simulink model "Thermal_Network_Model"  (R2022b)
settings: Solver=VariableStepAuto  StartTime=0.0  StopTime=24*3600*1  FixedStep=1  RelTol=1e-3  AbsTol=1e-3  EnableMultiTasking=on
InitFcn:
  | % Roof
  | roofArea =  2* (widHouse/(2*cos(pitRoof))*lenHouse);
  | 
  | %Rooms
  | %% Room 1
  | area_window_room1 = 3 * 1 *1;
  | area_wall_room1 = (lenHouse*3/5 *htHouse+widHouse*2/3*htHouse) - area_window_room1;
  | area_roof_room1 = roofArea/4;
  | 
  | %% Room 2
  | area_window_room2 = 2 * 1 *1;
  | area_wall_room2 = (lenHouse*3/5*htHouse+widHouse/3*htHouse) - area_window_room2;
  | area_roof_room2 = roofArea/4;
  | 
  | %% Room 3
  | area_window_room3 =2* 1 *1;
  | area_wall_room3 = (lenHouse*2/5*htHouse+widHouse*2/3*htHouse) - area_window_room3;
  | area_roof_room3 = roofArea/4;
  | 
  | %% Room 4
  | area_window_room4 = 2 * 1 *1;
  | area_wall_room4 = (lenHouse*2/5*htHouse+widHouse/3*htHouse) - area_window_room4;
  | area_roof_room4 = roofArea/4;
  | 
  | % Cost estimation
  | % Assume the cost of natural gas is $8.50 per thousand cubic feet (Mcf): $8.50 per 1000 cf
  | % cost = $8.50/(1000 * 0.02831) m^3
  | cost = 8.50/(1000 * 0.02831);
  | % Natural gas density ~ 0.9 kg/m^3
  | NG_density = 0.9;
values from neighbouring files (symbols this model uses):
  airDensity = 1.025    [Model_inputs.m]
  htHouse = 2.6    [Model_inputs.m]
  LCavity = 0.014    [Model_inputs.m]
  lenHouse = 15    [Model_inputs.m]
  load = struct()    [Model_inputs.m]
  LRoof = 0.2    [Model_inputs.m]
  LWall = 0.25    [Model_inputs.m]
  LWindow = 0.004    [Model_inputs.m]
  panel = struct()    [Model_inputs.m]
  pipe = struct()    [Model_inputs.m]
  pitRoof = 40/180/pi    (= 0.0707355302631)    [Model_inputs.m]
  roofDensity = 2440    [Model_inputs.m]
  tank = struct()    [Model_inputs.m]
  temp_initial = 20    [Model_inputs.m]
  wallDensity = 2400    [Model_inputs.m]
  widHouse = 8    [Model_inputs.m]
  windowDensity = 2500    [Model_inputs.m]
libraries: fl_lib x188, nesl_utility x51, SimscapeFluids_lib x14, fuzblock x6, ee_lib x1
(part 2 of 4)

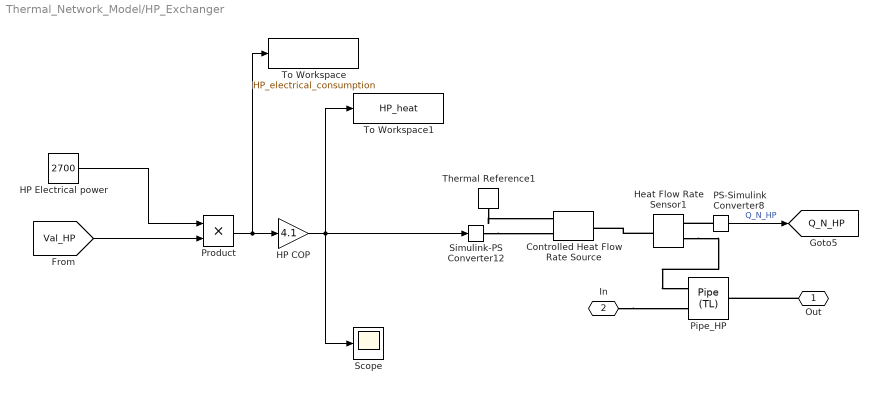
== system Thermal_Network_Model/HP_Exchanger ==
  Controlled Heat Flow Rate Source : fl_lib/Thermal/Thermal Sources/Controlled Heat Flow Rate Source
  HP COP : Gain  Gain=4.1
  HP Electrical power : Constant  Value=2700
  Heat Flow Rate Sensor1 : fl_lib/Thermal/Thermal Sensors/Heat Flow Rate Sensor
  PS-Simulink Converter8 : nesl_utility/PS-Simulink Converter  PhysicalDomain=network_engine_domain  SubClassName=ps_output  LeftPortType=input  RightPortType=output  PseudoPeriodic=off  Frequencies=[]  VectorFormat=1-D array  Unit=inherit  AffineConversion=off
  Pipe_HP : fl_lib/Thermal Liquid/Elements/Pipe (TL)  length=pipe.length m  area=pipe.area m^2  Dh=pipe.Dh m  length_add=pipe.length_add m  roughness=pipe.roughness m  Re_lam=pipe.Re_lam  Re_tur=pipe.Re_tur  shape_factor=pipe.shape_factor  Nu_lam=pipe.Nu_lam  dynamic_compressibility=simscape.enum.onoff.off  inertia=simscape.enum.onoff.off  p0=0.101325 MPa  T0=panel.initial.Tw0 K  mdot0=0 kg/s
  Product : Product
  Scope : Scope
  Simulink-PS Converter12 : nesl_utility/Simulink-PS Converter  PhysicalDomain=network_engine_domain  SubClassName=ps_input  LeftPortType=input  RightPortType=output  PseudoPeriodic=off  Frequencies=[]  NoiseDistribution=none  NoiseParameters=[]  Unit=1  AffineConversion=off  FilteringAndDerivatives=provide  SimscapeFilterOrder=1  InputFilterTimeConstant=0.001  UdotUserProvided=0
  Thermal Reference1 : fl_lib/Thermal/Thermal Elements/Thermal Reference
  To Workspace : ToWorkspace  VariableName=HP_electrical_consumption  SaveFormat=Timeseries  SampleTime=60
  To Workspace1 : ToWorkspace  VariableName=HP_heat  SaveFormat=Timeseries  SampleTime=60
  Out : PMIOPort  Side=Left
  In : PMIOPort  Port=2  Side=Right
  tag scope: Q_N_HP=global
  wires:
  PS-Simulink Converter8/1 -> [Q_N_HP]  "Q_N_HP"
  Product/1 -> To Workspace/1, HP COP/1
  [Val_HP] -> Product/2
  HP COP/1 -> Simulink-PS Converter12/1, Scope/1, To Workspace1/1
  HP Electrical power/1 -> Product/1
  connections:
  Heat Flow Rate Sensor1/RConn2 -- Pipe_HP/LConn2
  Thermal Reference1/LConn1 -- Controlled Heat Flow Rate Source/RConn2
  Heat Flow Rate Sensor1/LConn1 -- Controlled Heat Flow Rate Source/LConn1
  PS-Simulink Converter8/LConn1 -- Heat Flow Rate Sensor1/RConn1
  Simulink-PS Converter12/RConn1 -- Controlled Heat Flow Rate Source/RConn1
  Out/RConn1 -- Pipe_HP/RConn1
  In/RConn1 -- Pipe_HP/LConn1

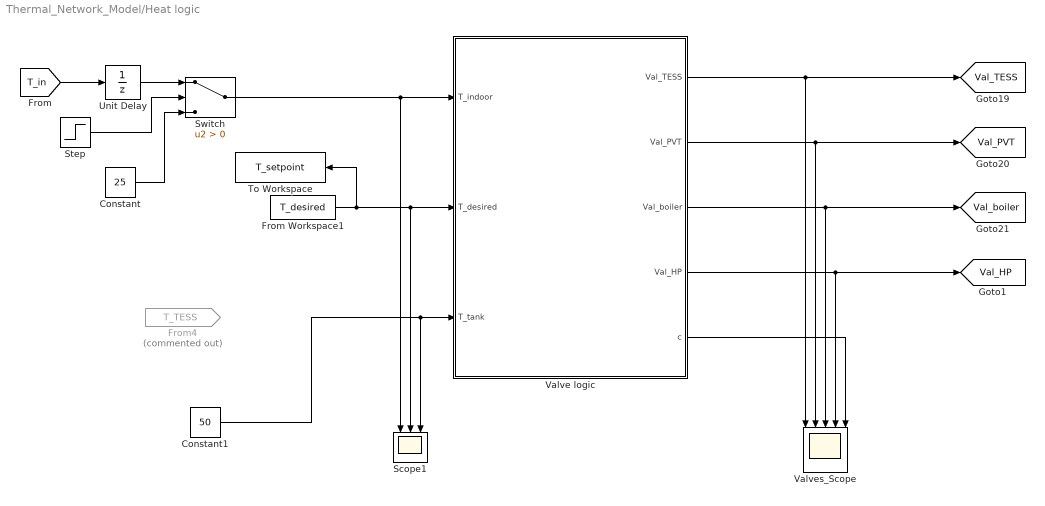
== system Thermal_Network_Model/Heat logic ==
  Constant : Constant  Value=25
  Constant1 : Constant  Value=50
  From Workspace1 : FromWorkspace  VariableName=T_desired
  From4 : From  Commented=on  GotoTag=T_TESS  TagVisibility=global
  Scope1 : Scope  NumInputPorts=3
  Step : Step  Time=3600  SampleTime=0
  Switch : Switch  Criteria=u2 > Threshold  SaturateOnIntegerOverflow=off  InputSameDT=off
  To Workspace : ToWorkspace  VariableName=T_setpoint  SaveFormat=Timeseries  SampleTime=-1
  Unit Delay : UnitDelay  SampleTime=-1  HasFrameUpgradeWarning=on
  Valve logic : MATLAB Function  TreatAsAtomicUnit=on
  Valves_Scope : Scope  NumInputPorts=5
  tag scope: Val_HP=global, Val_PVT=global, Val_TESS=global, Val_boiler=global
  wires:
  From Workspace1/1 -> To Workspace/1, Scope1/2, Valve logic/2(T_desired)
  Valve logic/1(Val_TESS) -> [Val_TESS], Valves_Scope/1
  Valve logic/2(Val_PVT) -> [Val_PVT], Valves_Scope/2
  Valve logic/3(Val_boiler) -> [Val_boiler], Valves_Scope/3
  Valve logic/4(Val_HP) -> [Val_HP], Valves_Scope/4
  Constant/1 -> Switch/3
  Step/1 -> Switch/2
  Switch/1 -> Scope1/1, Valve logic/1(T_indoor)
  [T_in] -> Unit Delay/1
  Unit Delay/1 -> Switch/1
  Valve logic/5(c) -> Valves_Scope/5
  Constant1/1 -> Valve logic/3(T_tank), Scope1/3

== system Thermal_Network_Model/House thermal network1 ==
  T_atm : Inport
  Indoor average temperature : Subsystem
  Radiator1 : Subsystem
      mask Display: disp('Radiator')
  Radiator2 : Subsystem
      mask Display: disp('Radiator')
  Radiator3 : Subsystem
      mask Display: disp('Radiator')
  Radiator4 : Subsystem
      mask Display: disp('Radiator')
  Room 1 : Subsystem  Tag=PublishSubsystem
      mask Display: disp('Room 1')
  Room 2 : Subsystem  Tag=PublishSubsystem
      mask Display: disp('Room 2')
  Room 3 : Subsystem  Tag=PublishSubsystem
      mask Display: disp('Room 3')
  Room 4 : Subsystem  Tag=PublishSubsystem
      mask Display: disp('Room 4')
  In : PMIOPort  Side=Left
  Out : PMIOPort  Port=2  Side=Left
  T_avg : Outport  VectorParamsAs1DForOutWhenUnconnected=off
  wires:
  T_atm/1 -> Room 1/1(Tatm), Room 2/1(Tatm), Room 3/1(Tatm), Room 4/1(Tatm)
  Indoor average temperature/1(T_avg) -> T_avg/1
  Room 2/1(Troom2) -> Indoor average temperature/3(T2)
  Room 4/1(Troom4) -> Indoor average temperature/1(T4)
  Room 3/1(Troom3) -> Indoor average temperature/2(T3)
  Room 1/1(Troom1) -> Indoor average temperature/4(T1)
  connections:
  Room 1/LConn1 -- Radiator1/LConn2
  Room 4/LConn1 -- Radiator4/LConn2
  Room 2/LConn1 -- Radiator2/LConn2
  Room 3/LConn1 -- Radiator3/LConn2
  Radiator1/RConn1 -- Out/RConn1 -- Radiator4/RConn1 -- Radiator3/RConn1 -- Radiator2/RConn1
  Radiator3/LConn1 -- Radiator2/LConn1 -- In/RConn1 -- Radiator1/LConn1 -- Radiator4/LConn1

== system Thermal_Network_Model/Network_Measures ==
  Absolute Reference (TL)2 : fl_lib/Thermal Liquid/Elements/Absolute Reference (TL)
  Density : Gain  Gain=1000
  PS-Simulink Converter5 : nesl_utility/PS-Simulink Converter  PhysicalDomain=network_engine_domain  SubClassName=ps_output  LeftPortType=input  RightPortType=output  PseudoPeriodic=off  Frequencies=[]  VectorFormat=1-D array  Unit=inherit  AffineConversion=off
  PS-Simulink Converter6 : nesl_utility/PS-Simulink Converter  PhysicalDomain=network_engine_domain  SubClassName=ps_output  LeftPortType=input  RightPortType=output  PseudoPeriodic=off  Frequencies=[]  VectorFormat=1-D array  Unit=inherit  AffineConversion=off
  PS-Simulink Converter7 : nesl_utility/PS-Simulink Converter  PhysicalDomain=network_engine_domain  SubClassName=ps_output  LeftPortType=input  RightPortType=output  PseudoPeriodic=off  Frequencies=[]  VectorFormat=1-D array  Unit=inherit  AffineConversion=off
  Pressure & Temperature Sensor (TL)2 : fl_lib/Thermal Liquid/Sensors/Pressure & Temperature Sensor (TL)
      settings: InternalSimscapePortConfiguration="{\"Bottom\":[],\"Left\":[{\"id\":\"A\",\"label\":\"A\",\"type\":\"foundation.thermal_liquid.thermal_liquid\"}],\"Right\":[{\"id\":\"B\",\"label\":\"B\",\"type\":\"foundation.thermal_liquid.thermal_liquid\"},{\"id\":\"P\",\"label\":\"P\",\"type\":\"output\"},{\"id\":\"T\",\"label\":\"T\",\"type\":\"output\"}],\"Top\":[]}"
  Volumetric Flow Rate Sensor (TL)1 : fl_lib/Thermal Liquid/Sensors/Volumetric Flow Rate Sensor (TL)
      settings: InternalSimscapePortConfiguration="{\"Bottom\":[],\"Left\":[{\"id\":\"A\",\"label\":\"A\",\"type\":\"foundation.thermal_liquid.thermal_liquid\"}],\"Right\":[{\"id\":\"B\",\"label\":\"B\",\"type\":\"foundation.thermal_liquid.thermal_liquid\"},{\"id\":\"V\",\"label\":\"V\",\"type\":\"output\"}],\"Top\":[]}"
  Out : PMIOPort  Side=Left
  In : PMIOPort  Port=2  Side=Right
  tag scope: P_Network=global, T_Network=global, massflow_Network=global
  wires:
  PS-Simulink Converter5/1 -> Density/1
  PS-Simulink Converter7/1 -> [P_Network]  "P_Network"
  Density/1 -> [massflow_Network]  "massflow_Network"
  PS-Simulink Converter6/1 -> [T_Network]  "T_Network"
  connections:
  Absolute Reference (TL)2/LConn1 -- Pressure & Temperature Sensor (TL)2/RConn1
  PS-Simulink Converter6/LConn1 -- Pressure & Temperature Sensor (TL)2/RConn3
  Volumetric Flow Rate Sensor (TL)1/RConn1 -- Out/RConn1 -- Pressure & Temperature Sensor (TL)2/LConn1
  PS-Simulink Converter5/LConn1 -- Volumetric Flow Rate Sensor (TL)1/RConn2
  PS-Simulink Converter7/LConn1 -- Pressure & Temperature Sensor (TL)2/RConn2
  In/RConn1 -- Volumetric Flow Rate Sensor (TL)1/LConn1

== system Thermal_Network_Model/Network_Pump ==
  Angular Velocity Source : fl_lib/Mechanical/Mechanical Sources/Ideal Angular Velocity Source
  Constant : Constant
  Fixed-Displacement Pump (TL) : SimscapeFluids_lib/Thermal Liquid/Pumps & Motors/Fixed-Displacement Pump (TL)  loss_spec=1  displacement=2e-5 m^3/rad  omega_nominal=150 rad/s  p_nominal=1 bar  mu_nominal=0.9 cP  vol_eff_nominal=0.92  mech_eff_nominal=0.88  no_load_torque=0.05 N*m  p_diff_eff_TLU=[0.1, 1, 2.55] MPa  omega_eff_TLU=[25, 50, 100, 200, 300, 400] rad/s  vol_eff_TLU=[0.816, 0.908, 0.954, 0.977, 0.981, 0.984; 0.325, 0.663, 0.831, 0.916, 0.925, 0.946; 0.137, 0.568, 0.78, 0.892, 0.893, 0.910]  mech_eff_TLU=[0.996, 0.996, 0.996, 0.996, 0.996, 0.996; 0.988, 0.989, 0.989, 0.989, 0.989, 0.990; 0.981, 0.981, 0.982, 0.982, 0.983, 0.984]  p_diff_loss_TLU=[.1, 1, 2] MPa  omega_loss_TLU=[25, 50, 100, 200, 300, 400] rad/s  vol_loss_TLU=[.023, .023, .023, .023, .0285, .032; .0844, .0842, .0845, .084, .1125, .108; .1079, .108, .11, .108, .1605, .18] * 1e-3 m^3/s  mech_loss_TLU=[.002, .002, .002, .002, .002, .002; .0607, .0556, .0556, .0556, .0556, .0505; .1937, .1937, .1833, .1833, .1729, .1626] N*m  vol_eff_min=1e-3  vol_eff_max=1  mech_eff_min=1e-3  mech_eff_max=1  pressure_threshold=1e-3 MPa  omega_threshold=10 rad/s  area=0.01 m^2  quadrant_check=0  pump_mode_check=simscape.enum.assert.action.none
  Mechanical Rotational Reference : fl_lib/Mechanical/Rotational Elements/Mechanical Rotational Reference
  Mechanical Rotational Reference1 : fl_lib/Mechanical/Rotational Elements/Mechanical Rotational Reference
  Product : Product
  Simulink-PS Converter : nesl_utility/Simulink-PS Converter  PhysicalDomain=network_engine_domain  SubClassName=ps_input  LeftPortType=input  RightPortType=output  PseudoPeriodic=off  Frequencies=[]  NoiseDistribution=none  NoiseParameters=[]  Unit=rpm  AffineConversion=off  FilteringAndDerivatives=zero  SimscapeFilterOrder=1  InputFilterTimeConstant=0.001  UdotUserProvided=1
  speed : Constant  Value=150*30/pi
  In : PMIOPort  Side=Left
  Out : PMIOPort  Port=2  Side=Right
  wires:
  Constant/1 -> Product/1
  Product/1 -> Simulink-PS Converter/1
  speed/1 -> Product/2
  connections:
  Out/RConn1 -- Fixed-Displacement Pump (TL)/LConn2
  Fixed-Displacement Pump (TL)/LConn1 -- In/RConn1
  Simulink-PS Converter/RConn1 -- Angular Velocity Source/RConn1
  Mechanical Rotational Reference1/LConn1 -- Angular Velocity Source/RConn2
  Mechanical Rotational Reference/LConn1 -- Fixed-Displacement Pump (TL)/RConn2
  Angular Velocity Source/LConn1 -- Fixed-Displacement Pump (TL)/RConn1

== system Thermal_Network_Model/Network_Pump1 ==
  Angular Velocity Source : fl_lib/Mechanical/Mechanical Sources/Ideal Angular Velocity Source
  Constant : Constant
  Fixed-Displacement Pump (TL) : SimscapeFluids_lib/Thermal Liquid/Pumps & Motors/Fixed-Displacement Pump (TL)  loss_spec=1  displacement=2e-5 m^3/rad  omega_nominal=150 rad/s  p_nominal=1 bar  mu_nominal=0.9 cP  vol_eff_nominal=0.92  mech_eff_nominal=0.88  no_load_torque=0.05 N*m  p_diff_eff_TLU=[0.1, 1, 2.55] MPa  omega_eff_TLU=[25, 50, 100, 200, 300, 400] rad/s  vol_eff_TLU=[0.816, 0.908, 0.954, 0.977, 0.981, 0.984; 0.325, 0.663, 0.831, 0.916, 0.925, 0.946; 0.137, 0.568, 0.78, 0.892, 0.893, 0.910]  mech_eff_TLU=[0.996, 0.996, 0.996, 0.996, 0.996, 0.996; 0.988, 0.989, 0.989, 0.989, 0.989, 0.990; 0.981, 0.981, 0.982, 0.982, 0.983, 0.984]  p_diff_loss_TLU=[.1, 1, 2] MPa  omega_loss_TLU=[25, 50, 100, 200, 300, 400] rad/s  vol_loss_TLU=[.023, .023, .023, .023, .0285, .032; .0844, .0842, .0845, .084, .1125, .108; .1079, .108, .11, .108, .1605, .18] * 1e-3 m^3/s  mech_loss_TLU=[.002, .002, .002, .002, .002, .002; .0607, .0556, .0556, .0556, .0556, .0505; .1937, .1937, .1833, .1833, .1729, .1626] N*m  vol_eff_min=1e-3  vol_eff_max=1  mech_eff_min=1e-3  mech_eff_max=1  pressure_threshold=1e-3 MPa  omega_threshold=10 rad/s  area=0.01 m^2  quadrant_check=0  pump_mode_check=simscape.enum.assert.action.none
  Mechanical Rotational Reference : fl_lib/Mechanical/Rotational Elements/Mechanical Rotational Reference
  Mechanical Rotational Reference1 : fl_lib/Mechanical/Rotational Elements/Mechanical Rotational Reference
  Product : Product
  Simulink-PS Converter : nesl_utility/Simulink-PS Converter  PhysicalDomain=network_engine_domain  SubClassName=ps_input  LeftPortType=input  RightPortType=output  PseudoPeriodic=off  Frequencies=[]  NoiseDistribution=none  NoiseParameters=[]  Unit=rpm  AffineConversion=off  FilteringAndDerivatives=zero  SimscapeFilterOrder=1  InputFilterTimeConstant=0.001  UdotUserProvided=1
  speed : Constant  Value=150*30/pi
  In : PMIOPort  Side=Left
  Out : PMIOPort  Port=2  Side=Right
  wires:
  speed/1 -> Product/2
  Product/1 -> Simulink-PS Converter/1
  Constant/1 -> Product/1
  connections:
  Angular Velocity Source/LConn1 -- Fixed-Displacement Pump (TL)/RConn1
  Mechanical Rotational Reference/LConn1 -- Fixed-Displacement Pump (TL)/RConn2
  Mechanical Rotational Reference1/LConn1 -- Angular Velocity Source/RConn2
  Simulink-PS Converter/RConn1 -- Angular Velocity Source/RConn1
  Fixed-Displacement Pump (TL)/LConn1 -- In/RConn1
  Out/RConn1 -- Fixed-Displacement Pump (TL)/LConn2

== system Thermal_Network_Model/Network_fluid ==
  Network_Tank : Scope
  PS-Simulink Converter8 : nesl_utility/PS-Simulink Converter  PhysicalDomain=network_engine_domain  SubClassName=ps_output  LeftPortType=input  RightPortType=output  PseudoPeriodic=off  Frequencies=[]  VectorFormat=1-D array  Unit=inherit  AffineConversion=off
  Tank3 : SimscapeFluids_lib/Thermal Liquid/Tanks & Accumulators/Tank (TL)  num_inlet=fluids.thermal_liquid.tanks_accumulators.enum.NumInlet.Two  pressure_spec=foundation.enum.pressure_spec.atmospheric  tank_pressure=0.101325 MPa  volume_spec=fluids.thermal_liquid.tanks_accumulators.enum.TankVolumeSpec.Constant  tank_area=0.5 m^2  level_TLU=[0, 3, 5] m  volume_TLU=[0, 4, 6] m^3  inlet_height_A=[.1] m  inlet_area_A=[.01] m^2  inlet_heights_AB=[0.1,0.1] m  inlet_areas_AB=[pipe.area,pipe.area] m^2  inlet_heights_ABC=[.1, .05, 0] m  inlet_areas_ABC=[.01, .01, .01] m^2  inlet_heights_ABCD=linspace(0.1, 0, 4) m  inlet_areas_ABCD=0.01 * ones(1, 4) m^2  inlet_heights_ABCDE=linspace(0.1, 0, 5) m  inlet_areas_ABCDE=0.01 * ones(1, 5) m^2  inlet_heights_ABCDEF=linspace(0.1, 0, 6) m  inlet_areas_ABCDEF=0.01 * ones(1, 6) m^2  level_check=simscape.enum.assert.action.error  capacity_check=simscape.enum.assert.action.warn  max_capacity=0.25 m^3  g=9.81 m/s^2  level_specify=on  level_priority=Low  level=0.25 m  level_nominal_specify=off  level_nominal_unit=m  level_nominal_value=1  volume_specify=on  volume_priority=Low  volume=0.25*0.5 m^3  volume_nominal_specify=off  volume_nominal_unit=m^3  volume_nominal_value=1  mass_specify=on  mass_priority=Low  mass=0.25*0.5*1000 kg  mass_nominal_specify=off  mass_nominal_unit=kg  mass_nominal_value=1  T_I_specify=on  T_I_priority=Low  T_I=tank.Ttank0 K  T_I_nominal_specify=off  T_I_nominal_unit=K  T_I_nominal_value=1
      settings: InternalSimscapePortConfiguration="{\"Bottom\":[{\"id\":\"H\",\"label\":\"H\",\"type\":\"foundation.thermal.thermal\"},{\"id\":\"T_out\",\"label\":\"T\",\"type\":\"output\"}],\"Left\":[{\"id\":\"A\",\"label\":\"A\",\"type\":\"foundation.thermal_liquid.thermal_liquid\"},{\"id\":\"B\",\"label\":\"B\",\"type\":\"foundation.thermal_liquid.thermal_liquid\"}],\"Right\":[],\"Top\":[{\"id\":\"V_out\",\"label\":\"V\",\"type\":\"output\"},{\"id\":\"L_out\",\"label\":\"L\",\"type\":\"output\"}]}"
  In : PMIOPort  Side=Left
  Out : PMIOPort  Port=2  Side=Right
  wires:
  PS-Simulink Converter8/1 -> Network_Tank/1  "Network_fluid_level"
  connections:
  In/RConn1 -- Tank3/LConn1
  PS-Simulink Converter8/LConn1 -- Tank3/LConn4
  Tank3/LConn2 -- Out/RConn1

== system Thermal_Network_Model/Optical model ==
  From Workspace : FromWorkspace  VariableName=Global_irradiation
  From Workspace1 : FromWorkspace  VariableName=Inclination_angle
  Goto3 : Goto  TagVisibility=global
  MATLAB Function : MATLAB Function  TreatAsAtomicUnit=on
  Product1 : Product
  Sum : Sum  Inputs=+-
  Unit Delay : UnitDelay  SampleTime=-1  HasFrameUpgradeWarning=on
  tag scope: C=global, D=global, E=global, P=global, S=global
  wires:
  MATLAB Function/1(Ir) -> [C]
  Sum/1 -> [E]
  MATLAB Function/2(heatg) -> [D]
  MATLAB Function/3(powAbspv) -> Sum/1
  Product1/1 -> Unit Delay/1
  [I] -> Product1/1
  [V] -> Product1/2
  From Workspace/1 -> [S], MATLAB Function/1(S)
  From Workspace1/1 -> MATLAB Function/2(Incl), Goto3/1
  Unit Delay/1 -> Sum/2, [P]

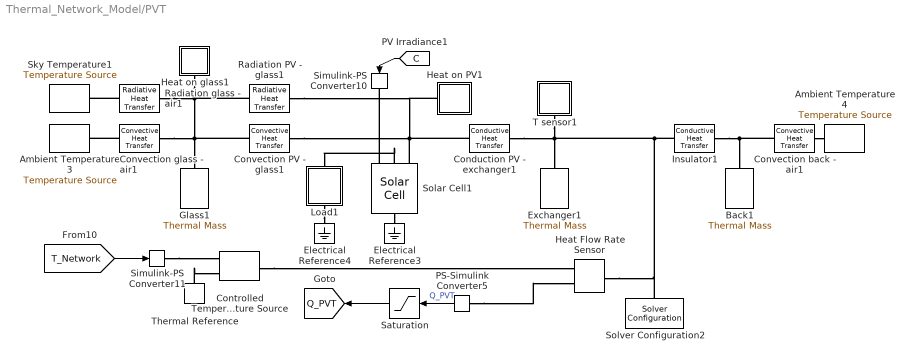
== system Thermal_Network_Model/PVT ==
  Ambient Temperature 3 : fl_lib/Thermal/Thermal Sources/Temperature Source  temperature=panel.heatTransfer.Ta K
  Ambient Temperature 4 : fl_lib/Thermal/Thermal Sources/Temperature Source  temperature=panel.heatTransfer.Ta K
  Back1 : fl_lib/Thermal/Thermal Elements/Thermal Mass  mass=panel.heatTransfer.Mb kg  sp_heat=panel.heatTransfer.Cb J/kg/K  num_ports=foundation.enum.numPorts2.one  T_specify=on  T_priority=High  T=panel.initial.Tb0 K  T_nominal_specify=off  T_nominal_unit=K  T_nominal_value=1  Q_specify=off  Q_priority=None  Q=0 W  Q_nominal_specify=off  Q_nominal_unit=W  Q_nominal_value=1
  Conduction PV - exchanger1 : fl_lib/Thermal/Thermal Elements/Conductive Heat Transfer  thermal_type=foundation.enum.ConstantVariableTabulated.Constant  wall_geometry=foundation.enum.ConductionWallGeometry.Planar  area=panel.geometry.Ncell*panel.geometry.Acell m^2  thickness=panel.heatTransfer.Le m  d_in=0.05 m  d_out=0.1 m  L=1 m  th_cond_min=10 W/(K*m)  th_cond=panel.heatTransfer.ke W/(m*K)  th_cond_TLU=[413, 401, 392, 383, 371, 357, 342] W/(K*m)  temp_TLU=[200, 273, 400, 600, 800, 1000, 1200] K  T_specify=off  T_priority=None  T=0 K  T_nominal_specify=off  T_nominal_unit=K  T_nominal_value=1  Q_specify=off  Q_priority=None  Q=0 W  Q_nominal_specify=off  Q_nominal_unit=W  Q_nominal_value=1
  Controlled Temperature Source : fl_lib/Thermal/Thermal Sources/Controlled Temperature Source
  Convection PV - glass1 : fl_lib/Thermal/Thermal Elements/Convective Heat Transfer  thermal_type=foundation.enum.constant_variable.constant  area=panel.geometry.Ncell*panel.geometry.Acell m^2  heat_tr_coeff=panel.heatTransfer.hgpv W/(m^2 * K)  min_heat_tr_coeff=1e-3 W/(K*m^2)  T_specify=off  T_priority=None  T=0 K  T_nominal_specify=off  T_nominal_unit=K  T_nominal_value=1  Q_specify=off  Q_priority=None  Q=0 W  Q_nominal_specify=off  Q_nominal_unit=W  Q_nominal_value=1
  Convection back - air1 : fl_lib/Thermal/Thermal Elements/Convective Heat Transfer  thermal_type=foundation.enum.constant_variable.constant  area=panel.geometry.Ncell*panel.geometry.Acell m^2  heat_tr_coeff=panel.heatTransfer.hba W/(m^2 * K)  min_heat_tr_coeff=1e-3 W/(K*m^2)  T_specify=off  T_priority=None  T=0 K  T_nominal_specify=off  T_nominal_unit=K  T_nominal_value=1  Q_specify=off  Q_priority=None  Q=0 W  Q_nominal_specify=off  Q_nominal_unit=W  Q_nominal_value=1
  Convection glass - air1 : fl_lib/Thermal/Thermal Elements/Convective Heat Transfer  thermal_type=foundation.enum.constant_variable.constant  area=panel.geometry.Ncell*panel.geometry.Acell m^2  heat_tr_coeff=panel.heatTransfer.hgpv W/(m^2 * K)  min_heat_tr_coeff=1e-3 W/(K*m^2)  T_specify=off  T_priority=None  T=0 K  T_nominal_specify=off  T_nominal_unit=K  T_nominal_value=1  Q_specify=off  Q_priority=None  Q=0 W  Q_nominal_specify=off  Q_nominal_unit=W  Q_nominal_value=1
  Electrical Reference3 : fl_lib/Electrical/Electrical Elements/Electrical Reference
  Electrical Reference4 : fl_lib/Electrical/Electrical Elements/Electrical Reference
  Exchanger1 : fl_lib/Thermal/Thermal Elements/Thermal Mass  mass=panel.heatTransfer.Me kg  sp_heat=panel.heatTransfer.Ce J/kg/K  num_ports=foundation.enum.numPorts2.one  T_specify=on  T_priority=High  T=panel.initial.Te0 K  T_nominal_specify=off  T_nominal_unit=K  T_nominal_value=1  Q_specify=off  Q_priority=None  Q=0 W  Q_nominal_specify=off  Q_nominal_unit=W  Q_nominal_value=1
  Glass1 : fl_lib/Thermal/Thermal Elements/Thermal Mass  mass=panel.heatTransfer.Mg kg  sp_heat=panel.heatTransfer.Cg J/kg/K  num_ports=foundation.enum.numPorts2.one  T_specify=on  T_priority=High  T=panel.initial.Tg0 K  T_nominal_specify=off  T_nominal_unit=K  T_nominal_value=1  Q_specify=off  Q_priority=None  Q=0 W  Q_nominal_specify=off  Q_nominal_unit=W  Q_nominal_value=1
  Heat Flow Rate Sensor : fl_lib/Thermal/Thermal Sensors/Heat Flow Rate Sensor
  Heat on PV1 : Subsystem
  Heat on glass1 : Subsystem
  Insulator1 : fl_lib/Thermal/Thermal Elements/Conductive Heat Transfer  thermal_type=foundation.enum.ConstantVariableTabulated.Constant  wall_geometry=foundation.enum.ConductionWallGeometry.Planar  area=panel.geometry.Ncell*panel.geometry.Acell m^2  thickness=panel.heatTransfer.Lins m  d_in=0.05 m  d_out=0.1 m  L=1 m  th_cond_min=10 W/(K*m)  th_cond=panel.heatTransfer.kins W/(m*K)  th_cond_TLU=[413, 401, 392, 383, 371, 357, 342] W/(K*m)  temp_TLU=[200, 273, 400, 600, 800, 1000, 1200] K  T_specify=off  T_priority=None  T=0 K  T_nominal_specify=off  T_nominal_unit=K  T_nominal_value=1  Q_specify=off  Q_priority=None  Q=0 W  Q_nominal_specify=off  Q_nominal_unit=W  Q_nominal_value=1
  Load1 : Subsystem
  PS-Simulink Converter5 : nesl_utility/PS-Simulink Converter  PhysicalDomain=network_engine_domain  SubClassName=ps_output  LeftPortType=input  RightPortType=output  PseudoPeriodic=off  Frequencies=[]  VectorFormat=1-D array  Unit=inherit  AffineConversion=off
  Radiation PV - glass1 : fl_lib/Thermal/Thermal Elements/Radiative Heat Transfer  area=panel.geometry.Ncell*panel.geometry.Acell m^2  rad_tr_coeff=5.670367e-8/(1/panel.heatTransfer.epsg + 1/panel.heatTransfer.epspv - 1) W/(m^2*K^4)  T_specify=off  T_priority=None  T=0 K  T_nominal_specify=off  T_nominal_unit=K  T_nominal_value=1  Q_specify=off  Q_priority=None  Q=0 W  Q_nominal_specify=off  Q_nominal_unit=W  Q_nominal_value=1
      settings: InternalSimscapePortConfiguration="{\"Bottom\":[],\"Left\":[{\"id\":\"A\",\"label\":\"A\",\"type\":\"foundation.thermal.thermal\"}],\"Right\":[{\"id\":\"B\",\"label\":\"B\",\"type\":\"foundation.thermal.thermal\"}],\"Top\":[]}"
  Radiation glass - air1 : fl_lib/Thermal/Thermal Elements/Radiative Heat Transfer  area=panel.geometry.Ncell*panel.geometry.Acell m^2  rad_tr_coeff=5.670367e-8*panel.heatTransfer.epsg W/(m^2*K^4)  T_specify=off  T_priority=None  T=0 K  T_nominal_specify=off  T_nominal_unit=K  T_nominal_value=1  Q_specify=off  Q_priority=None  Q=0 W  Q_nominal_specify=off  Q_nominal_unit=W  Q_nominal_value=1
      settings: InternalSimscapePortConfiguration="{\"Bottom\":[],\"Left\":[{\"id\":\"A\",\"label\":\"A\",\"type\":\"foundation.thermal.thermal\"}],\"Right\":[{\"id\":\"B\",\"label\":\"B\",\"type\":\"foundation.thermal.thermal\"}],\"Top\":[]}"
  Saturation : Saturate  UpperLimit=1000  LowerLimit=0
  Simulink-PS Converter10 : nesl_utility/Simulink-PS Converter  PhysicalDomain=network_engine_domain  SubClassName=ps_input  LeftPortType=input  RightPortType=output  PseudoPeriodic=off  Frequencies=[]  NoiseDistribution=none  NoiseParameters=[]  Unit=W/m^2  AffineConversion=off  FilteringAndDerivatives=provide  SimscapeFilterOrder=1  InputFilterTimeConstant=0.001  UdotUserProvided=0
  Simulink-PS Converter11 : nesl_utility/Simulink-PS Converter  PhysicalDomain=network_engine_domain  SubClassName=ps_input  LeftPortType=input  RightPortType=output  PseudoPeriodic=off  Frequencies=[]  NoiseDistribution=none  NoiseParameters=[]  Unit=1  AffineConversion=off  FilteringAndDerivatives=filter  SimscapeFilterOrder=1  InputFilterTimeConstant=0.001  UdotUserProvided=0
  Sky Temperature1 : fl_lib/Thermal/Thermal Sources/Temperature Source  temperature=panel.heatTransfer.Tsky K
  Solar Cell1 : ee_lib/Sources/Solar Cell  prm=1  Isc=panel.pv.Isc A  Voc=panel.pv.Voc V  Is=1e-6 A  Is2=0 A  Iph=7.34 A  Ir0=panel.pv.Ir0 W/m^2  ec=panel.pv.ec  N2=2  Rs=panel.pv.Rs Ohm  Rp=inf Ohm  N_series=panel.geometry.Ncell  N_parallel=1  TIPH1=panel.pv.TIPH1 1/K  EG=panel.pv.EG eV  TXIS1=panel.pv.TXIS1  TXIS2=3  TRS1=panel.pv.TRS1  TRP1=0  Tmeas=panel.pv.Tmeas degC  TFIXED=25 degC  thermal_mass=panel.heatTransfer.Mpv*panel.heatTransfer.Cpv J/K  initial_temperature=panel.initial.Tpv0 K
      settings: InternalSimscapePortConfiguration="{\"Bottom\":[],\"Left\":[{\"id\":\"Ir\",\"label\":\"Ir\",\"type\":\"input\"},{\"id\":\"p\",\"label\":\"+\",\"type\":\"foundation.electrical.electrical\"},{\"id\":\"H\",\"label\":\"H\",\"type\":\"foundation.thermal.thermal\"}],\"Right\":[{\"id\":\"n\",\"label\":\"-\",\"type\":\"foundation.electrical.electrical\"}],\"Top\":[]}"
  Solver Configuration2 : nesl_utility/Solver Configuration  PhysicalDomain=network_engine_domain  SubClassName=solver  LeftPortType=input  RightPortType=generic  Tones=[]  Harmonics=[]  SimulateNoise=off  Profile=off  UseLocalSampling=off  EnableSwitchedLinearOptims=on  FrequencyDomain=off  UseCCode=off  RelTol=0.001  AbsTol=1e-06  MinStep=1e-09  ToWorkspace=off  RevertToSquareIcSolve=off  NumHomotopyIterations=100  PhasorMode=off  PhasorModeNumHarmonics=1  ConsistencySolver=NEWTON_FTOL  IndexReductionMethod=DerivativeReplacement  DoDC=off  ResidualTolerance=1e-9  ConsistencyTolSource=GLOBAL  ConsistencyAbsTol=0.001  ConsistencyRelTol=0.001  ConsistencyTolFactor=0.001  UseLocalSolver=off  LocalSolverChoice=NE_BACKWARD_EULER_ADVANCER  ResolveIndetEquations=on  FunctionEvalNumThread=1  LocalSolverSampleTime=0.1  DoFixedCost=off  MaxNonlinIter=3  MaxModeIter=2  ComputeImpulses=off  ImpulseIterations=2  LinearAlgebra=auto  LinearAlgebraNumThread=0  EquationFormulation=NE_TIME_EF  DelaysMemoryBudget=1024  AutomaticFiltering=on  FilteringTimeConstant=0.001  PartitionStorageMethod=AS_NEEDED  PartitionMemoryBudget=1024  PartitionMethod=FAST
  T sensor1 : Subsystem
  Thermal Reference : fl_lib/Thermal/Thermal Elements/Thermal Reference
  tag scope: Q_PVT=global
  wires:
  PS-Simulink Converter5/1 -> Saturation/1  "Q_PVT"
  [C] -> Simulink-PS Converter10/1
  [T_Network] -> Simulink-PS Converter11/1
  Saturation/1 -> [Q_PVT]
  connections:
  Controlled Temperature Source/LConn1 -- Heat Flow Rate Sensor/RConn2
  Insulator1/LConn1 -- Heat Flow Rate Sensor/LConn1 -- Solver Configuration2/RConn1 -- T sensor1/LConn1 -- Conduction PV - exchanger1/RConn1 -- Exchanger1/LConn1
  Convection PV - glass1/LConn1 -- Solar Cell1/LConn3 -- Conduction PV - exchanger1/LConn1 -- Heat on PV1/LConn1 -- Radiation PV - glass1/LConn1
  PS-Simulink Converter5/LConn1 -- Heat Flow Rate Sensor/RConn1
  Thermal Reference/LConn1 -- Controlled Temperature Source/RConn2
  Radiation glass - air1/LConn1 -- Heat on glass1/LConn1 -- Radiation PV - glass1/RConn1 -- Glass1/LConn1 -- Convection PV - glass1/RConn1 -- Convection glass - air1/LConn1
  Insulator1/RConn1 -- Convection back - air1/LConn1 -- Back1/LConn1
  Load1/LConn1 -- Electrical Reference4/LConn1
  Convection back - air1/RConn1 -- Ambient Temperature 4/LConn1
  Solar Cell1/RConn1 -- Electrical Reference3/LConn1
  Convection glass - air1/RConn1 -- Ambient Temperature 3/LConn1
  Solar Cell1/LConn2 -- Load1/RConn1
  Solar Cell1/LConn1 -- Simulink-PS Converter10/RConn1
  Simulink-PS Converter11/RConn1 -- Controlled Temperature Source/RConn1
  Radiation glass - air1/RConn1 -- Sky Temperature1/LConn1

== system Thermal_Network_Model/PVT_Exchanger ==
  Controlled Heat Flow Rate Source : fl_lib/Thermal/Thermal Sources/Controlled Heat Flow Rate Source
  Heat Flow Rate Sensor1 : fl_lib/Thermal/Thermal Sensors/Heat Flow Rate Sensor
  PS-Simulink Converter8 : nesl_utility/PS-Simulink Converter  PhysicalDomain=network_engine_domain  SubClassName=ps_output  LeftPortType=input  RightPortType=output  PseudoPeriodic=off  Frequencies=[]  VectorFormat=1-D array  Unit=inherit  AffineConversion=off
  Pipe_PVT : fl_lib/Thermal Liquid/Elements/Pipe (TL)  length=pipe.length m  area=pipe.area m^2  Dh=pipe.Dh m  length_add=pipe.length_add m  roughness=pipe.roughness m  Re_lam=pipe.Re_lam  Re_tur=pipe.Re_tur  shape_factor=pipe.shape_factor  Nu_lam=pipe.Nu_lam  dynamic_compressibility=simscape.enum.onoff.off  inertia=simscape.enum.onoff.off  p0=0.101325 MPa  T0=panel.initial.Tw0 K  mdot0=0 kg/s
  Product : Product
  Simulink-PS Converter12 : nesl_utility/Simulink-PS Converter  PhysicalDomain=network_engine_domain  SubClassName=ps_input  LeftPortType=input  RightPortType=output  PseudoPeriodic=off  Frequencies=[]  NoiseDistribution=none  NoiseParameters=[]  Unit=1  AffineConversion=off  FilteringAndDerivatives=provide  SimscapeFilterOrder=1  InputFilterTimeConstant=0.001  UdotUserProvided=0
  Thermal Reference1 : fl_lib/Thermal/Thermal Elements/Thermal Reference
  Out : PMIOPort  Side=Left
  In : PMIOPort  Port=2  Side=Right
  tag scope: Q_N_PVT=global
  wires:
  [Q_PVT] -> Product/1
  [Val_PVT] -> Product/2
  PS-Simulink Converter8/1 -> [Q_N_PVT]  "Q_N_PVT"
  Product/1 -> Simulink-PS Converter12/1
  connections:
  Simulink-PS Converter12/RConn1 -- Controlled Heat Flow Rate Source/RConn1
  PS-Simulink Converter8/LConn1 -- Heat Flow Rate Sensor1/RConn1
  Out/RConn1 -- Pipe_PVT/RConn1
  Heat Flow Rate Sensor1/LConn1 -- Controlled Heat Flow Rate Source/LConn1
  Thermal Reference1/LConn1 -- Controlled Heat Flow Rate Source/RConn2
  Heat Flow Rate Sensor1/RConn2 -- Pipe_PVT/LConn2
  In/RConn1 -- Pipe_PVT/LConn1

== system Thermal_Network_Model/Scopes ==
  From7 : From  TagVisibility=global
  Outputs : Scope  NumInputPorts=5
  Solar variables : Scope  NumInputPorts=2
  wires:
  [P] -> Outputs/1
  [S] -> Solar variables/1
  From7/1 -> Solar variables/2
  [M] -> Outputs/5
  [W] -> Outputs/3
  [T] -> Outputs/4
  [F] -> Outputs/2

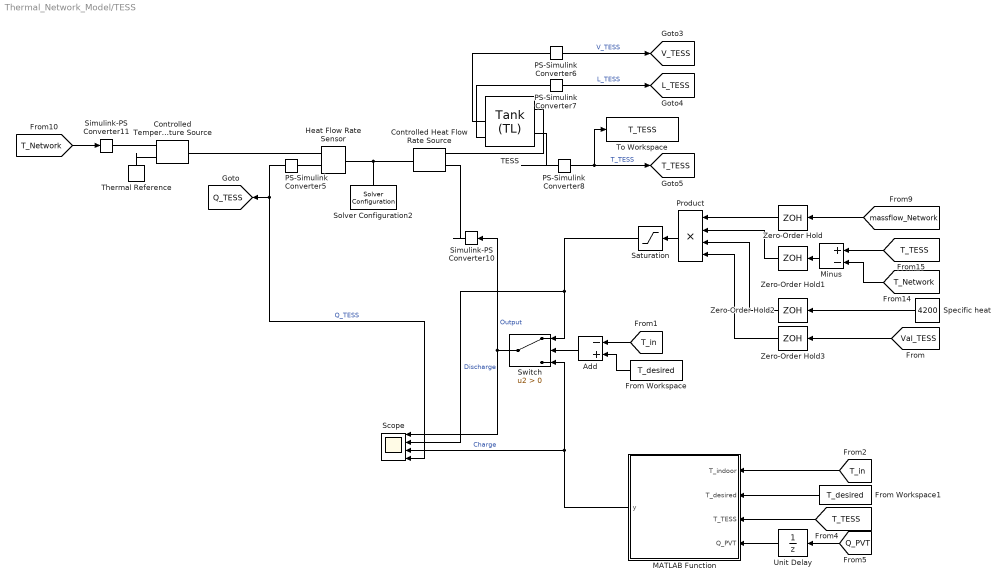
== system Thermal_Network_Model/TESS ==
  Add : Sum  Inputs=-+
  Controlled Temperature Source : fl_lib/Thermal/Thermal Sources/Controlled Temperature Source
  Controlled Heat Flow Rate Source : fl_lib/Thermal/Thermal Sources/Controlled Heat Flow Rate Source
  From Workspace : FromWorkspace  VariableName=T_desired
  From Workspace1 : FromWorkspace  VariableName=T_desired
  Heat Flow Rate Sensor : fl_lib/Thermal/Thermal Sensors/Heat Flow Rate Sensor
  MATLAB Function : MATLAB Function  TreatAsAtomicUnit=on
  Minus : Sum  Inputs=+-
  PS-Simulink Converter{5..8} (4 alike) : nesl_utility/PS-Simulink Converter  PhysicalDomain=network_engine_domain  SubClassName=ps_output  LeftPortType=input  RightPortType=output  PseudoPeriodic=off  Frequencies=[]  VectorFormat=1-D array  Unit=inherit  AffineConversion=off
  Product : Product  Inputs=4
  Saturation : Saturate  UpperLimit=1000  LowerLimit=-1000
  Scope : Scope  NumInputPorts=4
  Simulink-PS Converter10 : nesl_utility/Simulink-PS Converter  PhysicalDomain=network_engine_domain  SubClassName=ps_input  LeftPortType=input  RightPortType=output  PseudoPeriodic=off  Frequencies=[]  NoiseDistribution=none  NoiseParameters=[]  Unit=1  AffineConversion=off  FilteringAndDerivatives=provide  SimscapeFilterOrder=1  InputFilterTimeConstant=0.001  UdotUserProvided=0
  Simulink-PS Converter11 : nesl_utility/Simulink-PS Converter  PhysicalDomain=network_engine_domain  SubClassName=ps_input  LeftPortType=input  RightPortType=output  PseudoPeriodic=off  Frequencies=[]  NoiseDistribution=none  NoiseParameters=[]  Unit=1  AffineConversion=off  FilteringAndDerivatives=filter  SimscapeFilterOrder=1  InputFilterTimeConstant=0.001  UdotUserProvided=0
  Solver Configuration2 : nesl_utility/Solver Configuration  PhysicalDomain=network_engine_domain  SubClassName=solver  LeftPortType=input  RightPortType=generic  Tones=[]  Harmonics=[]  SimulateNoise=off  Profile=off  UseLocalSampling=off  EnableSwitchedLinearOptims=on  FrequencyDomain=off  UseCCode=off  RelTol=0.001  AbsTol=1e-06  MinStep=1e-09  ToWorkspace=off  RevertToSquareIcSolve=off  NumHomotopyIterations=100  PhasorMode=off  PhasorModeNumHarmonics=1  ConsistencySolver=NEWTON_FTOL  IndexReductionMethod=DerivativeReplacement  DoDC=off  ResidualTolerance=1e-9  ConsistencyTolSource=GLOBAL  ConsistencyAbsTol=0.001  ConsistencyRelTol=0.001  ConsistencyTolFactor=0.001  UseLocalSolver=off  LocalSolverChoice=NE_BACKWARD_EULER_ADVANCER  ResolveIndetEquations=on  FunctionEvalNumThread=1  LocalSolverSampleTime=0.1  DoFixedCost=off  MaxNonlinIter=3  MaxModeIter=2  ComputeImpulses=off  ImpulseIterations=2  LinearAlgebra=auto  LinearAlgebraNumThread=0  EquationFormulation=NE_TIME_EF  DelaysMemoryBudget=1024  AutomaticFiltering=on  FilteringTimeConstant=0.001  PartitionStorageMethod=AS_NEEDED  PartitionMemoryBudget=1024  PartitionMethod=FAST
  Specific heat : Constant  Value=4200
  Switch : Switch  Criteria=u2 > Threshold  SaturateOnIntegerOverflow=off  InputSameDT=off
  TESS : SimscapeFluids_lib/Thermal Liquid/Tanks & Accumulators/Tank (TL)  num_inlet=fluids.thermal_liquid.tanks_accumulators.enum.NumInlet.One  pressure_spec=foundation.enum.pressure_spec.atmospheric  tank_pressure=0.101325 MPa  volume_spec=fluids.thermal_liquid.tanks_accumulators.enum.TankVolumeSpec.Constant  tank_area=tank.Atank m^2  level_TLU=[0, 3, 5] m  volume_TLU=[0, 4, 6] m^3  inlet_height_A=[.1] m  inlet_area_A=[.01] m^2  inlet_heights_AB=[0.1,0.1] m  inlet_areas_AB=[pipe.area,pipe.area] m^2  inlet_heights_ABC=[.1, .05, 0] m  inlet_areas_ABC=[.01, .01, .01] m^2  inlet_heights_ABCD=linspace(0.1, 0, 4) m  inlet_areas_ABCD=0.01 * ones(1, 4) m^2  inlet_heights_ABCDE=linspace(0.1, 0, 5) m  inlet_areas_ABCDE=0.01 * ones(1, 5) m^2  inlet_heights_ABCDEF=linspace(0.1, 0, 6) m  inlet_areas_ABCDEF=0.01 * ones(1, 6) m^2  level_check=simscape.enum.assert.action.error  capacity_check=simscape.enum.assert.action.warn  max_capacity=tank.Volmax m^3  g=9.81 m/s^2  level_specify=on  level_priority=High  level=tank.Voltank0/tank.Atank m  level_nominal_specify=off  level_nominal_unit=m  level_nominal_value=1  volume_specify=off  volume_priority=High  volume=tank.Voltank0 m^3  volume_nominal_specify=off  volume_nominal_unit=m^3  volume_nominal_value=1  mass_specify=off  mass_priority=High  mass=tank.Voltank0*1000 kg  mass_nominal_specify=off  mass_nominal_unit=kg  mass_nominal_value=1  T_I_specify=on  T_I_priority=High  T_I=tank.Ttank0 K  T_I_nominal_specify=off  T_I_nominal_unit=K  T_I_nominal_value=1
      settings: InternalSimscapePortConfiguration="{\"Bottom\":[{\"id\":\"H\",\"label\":\"H\",\"type\":\"foundation.thermal.thermal\"},{\"id\":\"T_out\",\"label\":\"T\",\"type\":\"output\"}],\"Left\":[{\"id\":\"A\",\"label\":\"A\",\"type\":\"foundation.thermal_liquid.thermal_liquid\"}],\"Right\":[],\"Top\":[{\"id\":\"V_out\",\"label\":\"V\",\"type\":\"output\"},{\"id\":\"L_out\",\"label\":\"L\",\"type\":\"output\"}]}"
  Thermal Reference : fl_lib/Thermal/Thermal Elements/Thermal Reference
  To Workspace : ToWorkspace  VariableName=T_TESS  SaveFormat=Timeseries  SampleTime=-1
  Unit Delay : UnitDelay  SampleTime=-1  HasFrameUpgradeWarning=on
  Zero-Order Hold{,1..3} (4 alike) : ZeroOrderHold  SampleTime=10
  tag scope: L_TESS=global, Q_TESS=global, T_TESS=global, V_TESS=global
  wires:
  PS-Simulink Converter5/1 -> Scope/4, [Q_TESS]  "Q_TESS"
  Specific heat/1 -> Zero-Order Hold2/1
  [T_Network] -> Simulink-PS Converter11/1
  PS-Simulink Converter6/1 -> [V_TESS]  "V_TESS"
  [T_Network] -> Minus/2
  PS-Simulink Converter7/1 -> [L_TESS]  "L_TESS"
  [T_TESS] -> Minus/1
  [massflow_Network] -> Zero-Order Hold/1
  PS-Simulink Converter8/1 -> To Workspace/1, [T_TESS]  "T_TESS"
  [Val_TESS] -> Zero-Order Hold3/1
  Product/1 -> Saturation/1
  [T_in] -> Add/1
  From Workspace/1 -> Add/2
  Add/1 -> Switch/2
  Switch/1 -> Simulink-PS Converter10/1, Scope/1  "Output"
  Saturation/1 -> Scope/2, Switch/1  "Discharge"
  [T_in] -> MATLAB Function/1(T_indoor)
  From Workspace1/1 -> MATLAB Function/2(T_desired)
  [Q_PVT] -> Unit Delay/1
  [T_TESS] -> MATLAB Function/3(T_TESS)
  MATLAB Function/1(y) -> Scope/3, Switch/3  "Charge"
  Unit Delay/1 -> MATLAB Function/4(Q_PVT)
  Zero-Order Hold/1 -> Product/1
  Minus/1 -> Zero-Order Hold1/1
  Zero-Order Hold1/1 -> Product/2
  Zero-Order Hold2/1 -> Product/3
  Zero-Order Hold3/1 -> Product/4
  connections:
  PS-Simulink Converter7/LConn1 -- TESS/LConn3
  PS-Simulink Converter6/LConn1 -- TESS/LConn2
  Simulink-PS Converter11/RConn1 -- Controlled Temperature Source/RConn1
  PS-Simulink Converter5/LConn1 -- Heat Flow Rate Sensor/RConn1
  Controlled Heat Flow Rate Source/RConn2 -- TESS/RConn1
  Solver Configuration2/RConn1 -- Controlled Heat Flow Rate Source/LConn1 -- Heat Flow Rate Sensor/LConn1
  Thermal Reference/LConn1 -- Controlled Temperature Source/RConn2
  Controlled Temperature Source/LConn1 -- Heat Flow Rate Sensor/RConn2
  PS-Simulink Converter8/LConn1 -- TESS/RConn2
  Simulink-PS Converter10/RConn1 -- Controlled Heat Flow Rate Source/RConn1

== system Thermal_Network_Model/TESS_Exchanger ==
  Controlled Heat Flow Rate Source : fl_lib/Thermal/Thermal Sources/Controlled Heat Flow Rate Source
  Heat Flow Rate Sensor1 : fl_lib/Thermal/Thermal Sensors/Heat Flow Rate Sensor
  PS-Simulink Converter8 : nesl_utility/PS-Simulink Converter  PhysicalDomain=network_engine_domain  SubClassName=ps_output  LeftPortType=input  RightPortType=output  PseudoPeriodic=off  Frequencies=[]  VectorFormat=1-D array  Unit=inherit  AffineConversion=off
  Pipe_TESS : fl_lib/Thermal Liquid/Elements/Pipe (TL)  length=pipe.length m  area=pipe.area m^2  Dh=pipe.Dh m  length_add=pipe.length_add m  roughness=pipe.roughness m  Re_lam=pipe.Re_lam  Re_tur=pipe.Re_tur  shape_factor=pipe.shape_factor  Nu_lam=pipe.Nu_lam  dynamic_compressibility=simscape.enum.onoff.off  inertia=simscape.enum.onoff.off  p0=0.101325 MPa  T0=panel.initial.Tw0 K  mdot0=0 kg/s
  Product : Product
  Saturation : Saturate  UpperLimit=1000  LowerLimit=-1000
  Simulink-PS Converter12 : nesl_utility/Simulink-PS Converter  PhysicalDomain=network_engine_domain  SubClassName=ps_input  LeftPortType=input  RightPortType=output  PseudoPeriodic=off  Frequencies=[]  NoiseDistribution=none  NoiseParameters=[]  Unit=1  AffineConversion=off  FilteringAndDerivatives=provide  SimscapeFilterOrder=1  InputFilterTimeConstant=0.001  UdotUserProvided=0
  Thermal Reference1 : fl_lib/Thermal/Thermal Elements/Thermal Reference
  Zero-Order Hold : ZeroOrderHold  SampleTime=10
  Out : PMIOPort  Side=Left
  In : PMIOPort  Port=2  Side=Right
  tag scope: Q_N_TESS=global
  wires:
  PS-Simulink Converter8/1 -> [Q_N_TESS]  "Q_N_TESS"
  Product/1 -> Saturation/1
  [Val_TESS] -> Product/2
  [Q_TESS] -> Product/1
  Saturation/1 -> Zero-Order Hold/1
  Zero-Order Hold/1 -> Simulink-PS Converter12/1
  connections:
  In/RConn1 -- Pipe_TESS/LConn1
  Heat Flow Rate Sensor1/RConn2 -- Pipe_TESS/LConn2
  Thermal Reference1/LConn1 -- Controlled Heat Flow Rate Source/RConn2
  Heat Flow Rate Sensor1/LConn1 -- Controlled Heat Flow Rate Source/LConn1
  Out/RConn1 -- Pipe_TESS/RConn1
  PS-Simulink Converter8/LConn1 -- Heat Flow Rate Sensor1/RConn1
  Simulink-PS Converter12/RConn1 -- Controlled Heat Flow Rate Source/RConn1

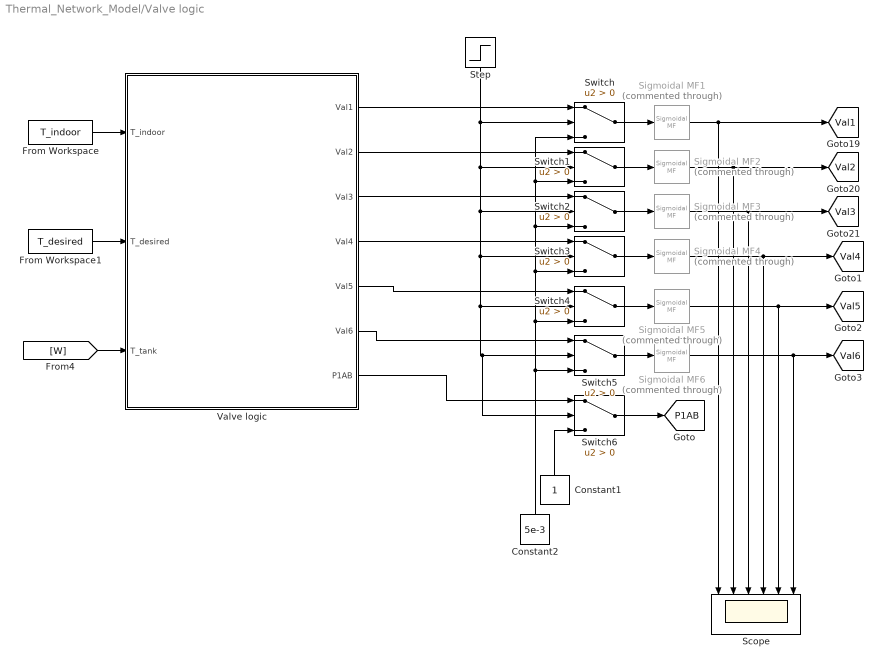
== system Thermal_Network_Model/Valve logic ==
  Constant1 : Constant
  Constant2 : Constant  Value=5e-3
  From Workspace : FromWorkspace  VariableName=T_indoor
  From Workspace1 : FromWorkspace  VariableName=T_desired
  Scope : Scope  NumInputPorts=6
  Sigmoidal MF{1..6} (6 alike) : fuzblock/Membership  Functions/Sigmoidal MF  Commented=through  a=30000  c=0
  Step : Step  SampleTime=0
  Switch{,1..6} (7 alike) : Switch  Criteria=u2 > Threshold  SaturateOnIntegerOverflow=off  InputSameDT=off
  Valve logic : MATLAB Function  TreatAsAtomicUnit=on
  tag scope: P1AB=global, Val1=global, Val2=global, Val3=global, Val4=global, Val5=global, Val6=global
  wires:
  Switch/1 -> Sigmoidal MF1/1
  Valve logic/1(Val1) -> Switch/1
  Step/1 -> Switch/2, Switch2/2, Switch3/2, Switch4/2, Switch6/2, Switch5/2, Switch1/2
  Valve logic/3(Val3) -> Switch2/1
  Constant2/1 -> Switch5/3, Switch4/3, Switch3/3, Switch2/3, Switch/3, Switch1/3
  [W] -> Valve logic/3(T_tank)
  Valve logic/2(Val2) -> Switch1/1
  Switch2/1 -> Sigmoidal MF3/1
  Switch1/1 -> Sigmoidal MF2/1
  Sigmoidal MF2/1 -> [Val2], Scope/2
  Sigmoidal MF1/1 -> [Val1], Scope/1
  Sigmoidal MF3/1 -> [Val3], Scope/3
  From Workspace/1 -> Valve logic/1(T_indoor)
  From Workspace1/1 -> Valve logic/2(T_desired)
  Sigmoidal MF4/1 -> [Val4], Scope/4
  Switch3/1 -> Sigmoidal MF4/1
  Valve logic/4(Val4) -> Switch3/1
  Valve logic/5(Val5) -> Switch4/1
  Valve logic/6(Val6) -> Switch5/1
  Switch4/1 -> Sigmoidal MF5/1
  Switch5/1 -> Sigmoidal MF6/1
  Sigmoidal MF5/1 -> Scope/5, [Val5]
  Sigmoidal MF6/1 -> [Val6], Scope/6
  Switch6/1 -> [P1AB]
  Valve logic/7(P1AB) -> Switch6/1
  Constant1/1 -> Switch6/3

== system Thermal_Network_Model/Boiler_Exchanger/Boiler ==
  mdot_fuel : Inport
  E-NTU Heat Exchanger (TL) : SimscapeFluids_lib/Fluid Network Interfaces/Heat Exchangers/Heat Exchanger (TL)  hex_type=1  shell_num=1  cross_type=1  NTU_TLU=[0.5, 1, 2, 3, 4, 5]  CR_TLU=[0, 0.25, 0.5, 0.75, 1]  eff_TLU=[0.30, 0.30, 0.30, 0.30, 0.30; 0.60, 0.55, 0.50, 0.47, 0.43; 0.85, 0.76, 0.68, 0.61, 0.55; 0.94, 0.83, 0.72, 0.65, 0.58; 0.98, 0.86, 0.75, 0.66, 0.58; 0.99, 0.86, 0.75, 0.66, 0.58]  R_wall=1.6e-4 K/W  min_flow_area_1=0.01 m^2  Dh_press_1=0.1 m  liquid_volume_1=0.01 m^3  Re_lam_1=2000  Re_tur_1=4000  pressure_loss_spec_1=1  pressure_loss_coeff_1=0.1  length_press_1=1 m  length_add_1=0.1 m  roughness_1=15e-6 m  Re_friction_TLU_1=[400, 1000, 1500, 3e3, 4e3, 6e3, 1e4, 2e4, 4e4, 6e4, 1e5, 1e8]  friction_factor_TLU_1=[0.264, 0.112, 0.071, 0.0417, 0.0387, 0.0268, 0.0250, 0.0232, 0.0226, 0.0220, 0.0214, 0.0214]  shape_factor_1=64  Re_Euler_TLU_1=[50, 500, 1000, 2000]  Euler_TLU_1=[4.4505, 0.6864, 0.4791, 0.3755]  heat_transfer_spec_1=1  heat_transfer_area_1=0.5 m^2  heat_coeff_1=500 W/(m^2 *K)  length_heat_1=1 m  Nu_lam_1=3.66  Re_Colburn_TLU_1=[100, 150, 1000]  Colburn_factor_TLU_1=[0.019, 0.013, 0.002]  Re_Nu_TLU_1=[100, 150, 1000]  Pr_Nu_TLU_1=[1, 10]  Nu_TLU_1=[3.72, 4.21; 3.75, 4.44; 4.21, 7.15]  fouling_factor_1=1e-4 m^2*K/W  min_heat_coeff_1=5 W/(m^2 * K)  heat_transfer_area_2=0.5 m^2  fouling_factor_2=1e-4 m^2*K/W  min_heat_coeff_2=0.01 W/(m^2 *K)  dynamic_compressibility_1=1  T0_1=300 K  p0_1=0.101325 MPa  mdot1_TLU=[.3, .5, .6, .7, 1, 1.4, 1.9, 2.3] kg/s  mdot2_TLU=[.3, .5, 1, 1.3, 1.7, 2, 2.6, 3.3] kg/s  SD_TLU=[.324, .3533, .404, .4253, .4333, .4373, .4453, .4533; .3813, .424, .496, .5307, .544, .5547, .5693, .5787; .4267, .4827, .5813, .6173, .6413, .6573, .672, .6827; .4613, .528, .64, .6987, .7267, .7467, .7707, .7853; .5533, .6467, .8227, .928, .9853, 1.0187, 1.0653, 1.0973; .58, .688, .8853, 1.0147, 1.08, 1.124, 1.176, 1.2147; .624, .7467, .992, 1.148, 1.244, 1.304, 1.3773, 1.4267; .656, .7907, 1.0667, 1.26, 1.376, 1.452, 1.548, 1.612] kW/K  Q_check=1  mdot_dp_TLU_1=[.3, .5, 1, 1.5, 2, 2.5] kg/s  p_diff_TLU_1=[3, 5, 10, 25, 35, 50] * 1e-3 MPa  T_ref_in_1=293.15 K  p_ref_in_1=0.101325 MPa  mdot_threshold_1=1e-3 kg/s  area_1=0.01 m^2
      settings: InternalSimscapePortConfiguration="{\"Bottom\":[],\"Left\":[{\"id\":\"A1\",\"label\":\"A1\",\"type\":\"foundation.thermal_liquid.thermal_liquid\"},{\"id\":\"B1\",\"label\":\"B1\",\"type\":\"foundation.thermal_liquid.thermal_liquid\"}],\"Right\":[{\"id\":\"H2\",\"label\":\"H2\",\"type\":\"foundation.thermal.thermal\"},{\"id\":\"C2\",\"label\":\"C2\",\"type\":\"input\"},{\"id\":\"HC2\",\"label\":\"HC2\",\"type\":\"input\"}],\"Top\":[]}"
  Furnace : SimscapeComponentBlock  SourceFile=furnace  ComponentPath=furnace  ComponentVariants=furnace  ComponentVariantNames=furnace  ClassName=furnace  SchemaVersion=1  excess_air=0.1  n=3.95  LHV=41e6 J/kg  cp_fuel=1880 J/kg/K  cp_air=1005 J/kg/K  cp_vapor=1820 J/kg/K  mdot_fuel_min=1e-5 kg/s
      settings: CopyFcn=simscape.engine.sli.internal.componentblockcallback(gcbh,'COPY')  PreCopyFcn=simscape.engine.sli.internal.componentblockcallback(gcbh,'PRECOPY')  PreDeleteFcn=simscape.engine.sli.internal.componentblockcallback(gcbh,'PREDELETE')  InternalSimscapePortConfiguration="{\"Bottom\":[],\"Left\":[{\"id\":\"Mdot_fuel\",\"label\":\"MF\",\"type\":\"input\"},{\"id\":\"T_fuel\",\"label\":\"TF\",\"type\":\"input\"},{\"id\":\"Humid_ratio\",\"label\":\"HR\",\"type\":\"input\"},{\"id\":\"T_air\",\"label\":\"TS\",\"type\":\"input\"}],\"Right\":[{\"id\":\"H\",\"label\":\"H\",\"type\":\"foundation.thermal.thermal\"},{\"id\":\"C_exh\",\"label\":\"C_exh\",\"type\":\"output\"}],\"Top\":[]}"
      mask Type: Furnace
  HC2 : fl_lib/Physical Signals/Sources/PS Constant  constant=500
  Humidity ratio : fl_lib/Physical Signals/Sources/PS Constant  constant=0.005
  Simulink-PS Converter : nesl_utility/Simulink-PS Converter  PhysicalDomain=network_engine_domain  SubClassName=ps_input  LeftPortType=input  RightPortType=output  PseudoPeriodic=off  Frequencies=[]  NoiseDistribution=none  NoiseParameters=[]  Unit=kg/s  AffineConversion=off  FilteringAndDerivatives=zero  SimscapeFilterOrder=1  InputFilterTimeConstant=0.001  UdotUserProvided=1
  T_air : fl_lib/Physical Signals/Sources/PS Constant  constant=15+273.15
  T_fuel : fl_lib/Physical Signals/Sources/PS Constant  constant=10+273.15
  Inlet : PMIOPort  Side=Left
  Outlet : PMIOPort  Port=2  Side=Right
  wires:
  mdot_fuel/1 -> Simulink-PS Converter/1
  connections:
  E-NTU Heat Exchanger (TL)/LConn2 -- Outlet/RConn1
  Furnace/LConn4 -- T_air/RConn1
  Furnace/LConn1 -- Simulink-PS Converter/RConn1
  Inlet/RConn1 -- E-NTU Heat Exchanger (TL)/LConn1
  Furnace/LConn3 -- Humidity ratio/RConn1
  Furnace/LConn2 -- T_fuel/RConn1
  Furnace/RConn1 -- E-NTU Heat Exchanger (TL)/RConn1
  Furnace/RConn2 -- E-NTU Heat Exchanger (TL)/RConn2
  HC2/RConn1 -- E-NTU Heat Exchanger (TL)/RConn3

== system Thermal_Network_Model/House thermal network1/Indoor average temperature ==
  T4 : Inport
  T3 : Inport  Port=2
  T2 : Inport  Port=3
  T1 : Inport  Port=4
  Add : Sum
  Constant : Constant  Value=0
  Gain : Gain  Gain=0.25
  Sum of Elements : Sum  Inputs=++++
  T_avg : Outport  VectorParamsAs1DForOutWhenUnconnected=off
  wires:
  Gain/1 -> Add/1
  Sum of Elements/1 -> Gain/1
  Add/1 -> T_avg/1
  Constant/1 -> Add/2
  T3/1 -> Sum of Elements/2
  T4/1 -> Sum of Elements/1
  T1/1 -> Sum of Elements/4
  T2/1 -> Sum of Elements/3
